simulink model "PID"  (R2024b)
settings: Solver=VariableStepAuto  StartTime=0.0  StopTime=75  RelTol=1e-3
settings Model: Creator=honor  LastModifiedBy=honor

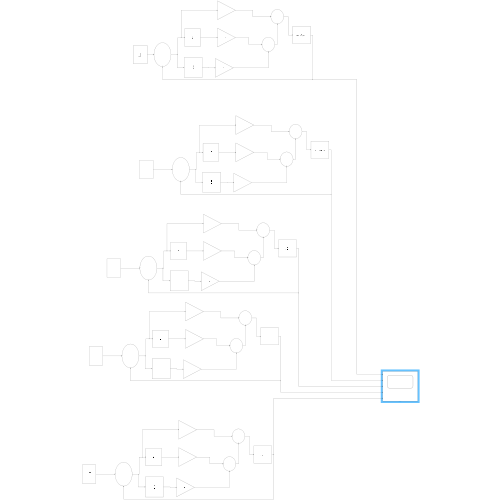
[thumbnail: Simulink's stored preview of the top-level diagram]
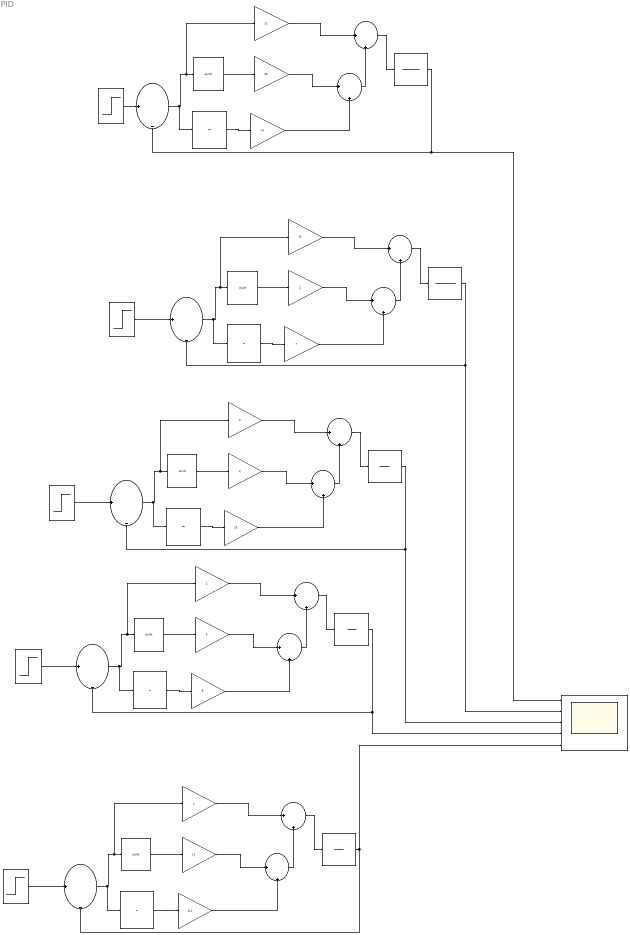
== system PID ==
  Derivative{,1..4} (5 alike) : Derivative
  Gain : Gain  Gain=14
  Gain1 : Gain  Gain=45
  Gain10 : Gain  Gain=5
  Gain11 : Gain  Gain=2
  Gain12 : Gain  Gain=111
  Gain13 : Gain  Gain=11
  Gain14 : Gain
  Gain2 : Gain  Gain=11
  Gain3 : Gain  Gain=7
  Gain4 : Gain  Gain=2
  Gain5 : Gain  Gain=15
  Gain6 : Gain  Gain=25
  Gain7 : Gain  Gain=2
  Gain8 : Gain  Gain=5
  Gain9 : Gain  Gain=8
  Integrator{,1..4} (5 alike) : Integrator
  Scope : Scope  NumInputPorts=5
  Step : Step  SampleTime=0.1
  Step1 : Step  After=2  SampleTime=0.1
  Step2 : Step  After=3  SampleTime=0.1
  Step3 : Step  After=4  SampleTime=0.1
  Step4 : Step  After=5  SampleTime=0.1
  Sum{,1,3..4,6..7,9..10,12..13} (10 alike) : Sum  Inputs=|++
  Sum{2,5,8,11,14} (5 alike) : Sum  Inputs=|+-
  Transfer Fcn : TransferFcn  Denominator=[19 19 8 1]
  Transfer Fcn1 : TransferFcn  Denominator=[12 32 43 54]
  Transfer Fcn2 : TransferFcn  Denominator=[ 2 5 8 ]
  Transfer Fcn3 : TransferFcn  Denominator=[1 2 7 ]
  Transfer Fcn4 : TransferFcn  Denominator=[1 4 9]
  wires:
  Derivative/1 -> Gain1/1
  Integrator/1 -> Gain/1
  Gain1/1 -> Sum/1
  Gain/1 -> Sum/2
  Gain2/1 -> Sum1/1
  Sum/1 -> Sum1/2
  Sum1/1 -> Transfer Fcn/1
  Step/1 -> Sum2/1
  Sum2/1 -> Integrator/1, Gain2/1, Derivative/1
  Transfer Fcn/1 -> Sum2/2, Scope/1
  Transfer Fcn1/1 -> Scope/2, Sum5/2
  Step1/1 -> Sum5/1
  Sum5/1 -> Integrator1/1, Gain5/1, Derivative1/1
  Gain5/1 -> Sum4/1
  Gain4/1 -> Sum3/1
  Derivative1/1 -> Gain4/1
  Gain3/1 -> Sum3/2
  Integrator1/1 -> Gain3/1
  Sum3/1 -> Sum4/2
  Sum4/1 -> Transfer Fcn1/1
  Step2/1 -> Sum8/1
  Sum7/1 -> Transfer Fcn2/1
  Gain8/1 -> Sum7/1
  Transfer Fcn2/1 -> Scope/3, Sum8/2
  Sum6/1 -> Sum7/2
  Integrator2/1 -> Gain6/1
  Gain6/1 -> Sum6/2
  Sum8/1 -> Integrator2/1, Gain8/1, Derivative2/1
  Derivative2/1 -> Gain7/1
  Gain7/1 -> Sum6/1
  Sum9/1 -> Sum10/2
  Transfer Fcn3/1 -> Scope/4, Sum11/2
  Integrator3/1 -> Gain9/1
  Gain9/1 -> Sum9/2
  Gain11/1 -> Sum10/1
  Sum11/1 -> Integrator3/1, Gain11/1, Derivative3/1
  Step3/1 -> Sum11/1
  Sum10/1 -> Transfer Fcn3/1
  Gain10/1 -> Sum9/1
  Derivative3/1 -> Gain10/1
  Sum12/1 -> Sum13/2
  Transfer Fcn4/1 -> Scope/5, Sum14/2
  Integrator4/1 -> Gain12/1
  Gain12/1 -> Sum12/2
  Gain14/1 -> Sum13/1
  Sum14/1 -> Integrator4/1, Gain14/1, Derivative4/1
  Step4/1 -> Sum14/1
  Sum13/1 -> Transfer Fcn4/1
  Gain13/1 -> Sum12/1
  Derivative4/1 -> Gain13/1
